simulink model "s7_template_extra"  (R2023a)
settings: Solver=ode4  StartTime=0.0  StopTime=inf  FixedStep=P_sim_dt  RelTol=1e-3
InitFcn:
  | s6_data
values from neighbouring files (symbols this model uses):
  breakslen = varargin{1}    [mbc_ppval.m]
  P_cx_k = 1    [s6_data.m]
  P_p_Bf = 0.7    [p_mad_car.m]
  P_p_Br = 0.7    [p_mad_car.m]
  P_p_Cf = 2    [p_mad_car.m]
  P_p_Cr = 2    [p_mad_car.m]
  P_p_delta_max = 21.58/180*pi    (= 0.37664205258)    [p_mad_car.m]
  P_p_Df = 2    [p_mad_car.m]
  P_p_Dr = 2.5    [p_mad_car.m]
  P_p_Ef = -0.1    [p_mad_car.m]
  P_p_Er = -0.05    [p_mad_car.m]
  P_p_J = 192e-6    (= 0.000192)    [p_mad_car.m]
  P_p_k = 2.51    [p_mad_car.m]
  P_p_kr = 0.344014    [s6_data.m]
  P_p_l = abs(P_p_frontaxle_1 + P_p_rearaxle_1)    [p_mad_car.m]
  P_p_lf = P_p_frontaxle_1    (= 0.05)    [p_mad_car.m]
  P_p_lr = P_p_rearaxle_1    (= 0.049)    [p_mad_car.m]
  P_p_m = 132e-3    (= 0.132)    [p_mad_car.m]
  P_p_T = 316e-3    (= 0.316)    [p_mad_car.m]
  P_p_TA = 0.02    [s6_data.m]
  P_p_Ti = 0.246830    (= 0.24683)    [s6_data.m]
  P_p_Tt = P_p_uTt + P_p_output_Tt    (= 0.1)    [p_mad_car.m]
  P_w_breakslen = uint32(length(path.points))    [s6_data.m]
  P_w_coefs = zeros(SPLINE.Elements(3).Dimensions)    [s6_data.m]
  P_w_points = zeros(SPLINE.Elements(2).Dimensions)    [s6_data.m]
  P_w_segments = uint32(zeros(SPLINE.Elements(4).Dimensions))    [s6_data.m]
  points = [ p.x + x ;      center1 + sign(t.xe) * r * cos(p.psi - pi/2 + sign(t.xe) * x / t.r) ;      center2 + sign(t.xe) * r * sin(p.psi - pi/2 + sign(t.xe) * x / t.r) ]    [mbc_circle_get_points.m]    (also in mbc_clothoid_get_points.m = [ p.x + x ;      s1;      s2]; mbc_spline_create.m = [ points(:, 1:end-1) [ points(1, end); points(2:3, 1) ] ]; mbc_straight_get_points.m = [ p.x + x ;      p.s1 + cpsi * x + (alpha - 0.5) * t.w * cos)
undefined symbols (not defined in the file or in its folder): coefs, DiscIntNeverNeededParam, Display, mad_lib_template, mbc_car_display, P_p_s1_start, P_p_s2_start, P_p_Tw, periodic, segments
settings Model: Creator=hmekiedj  LastModifiedBy=aaron
settings SolverCC: AlgebraicLoopSolver=TrustRegion
settings DataIOCC: ReturnWorkspaceOutputs=off
settings OptimizationCC: BlockReduction=off  DefaultParameterBehavior=Inlined  BufferReuse=off
settings DebuggingCC: SignalInfNanChecking=warning  UnconnectedInputMsg=warning  UnconnectedOutputMsg=warning  UnconnectedLineMsg=warning  ArithmeticOperatorsInVariantConditions=warning
settings ModelReferenceCC: EnableRefExpFcnMdlSchedulingChecks=on
settings SFSimCC: SimUseLocalCustomCode=off  CustomCodeUndefinedFunction=UseInterfaceOnly
settings RTWCC: RTWUseLocalCustomCode=off
settings CodeAppCC: StateflowObjectComments=on

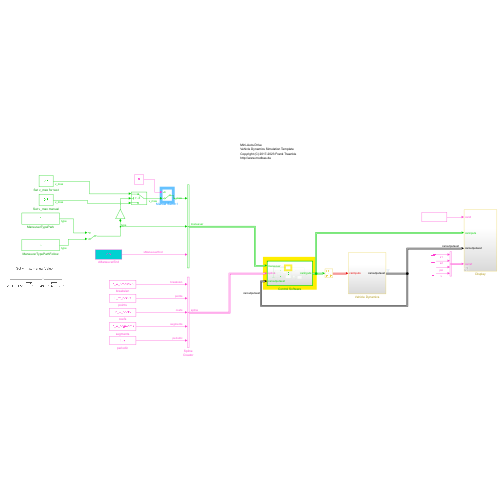
[thumbnail: Simulink's stored preview of the top-level diagram]
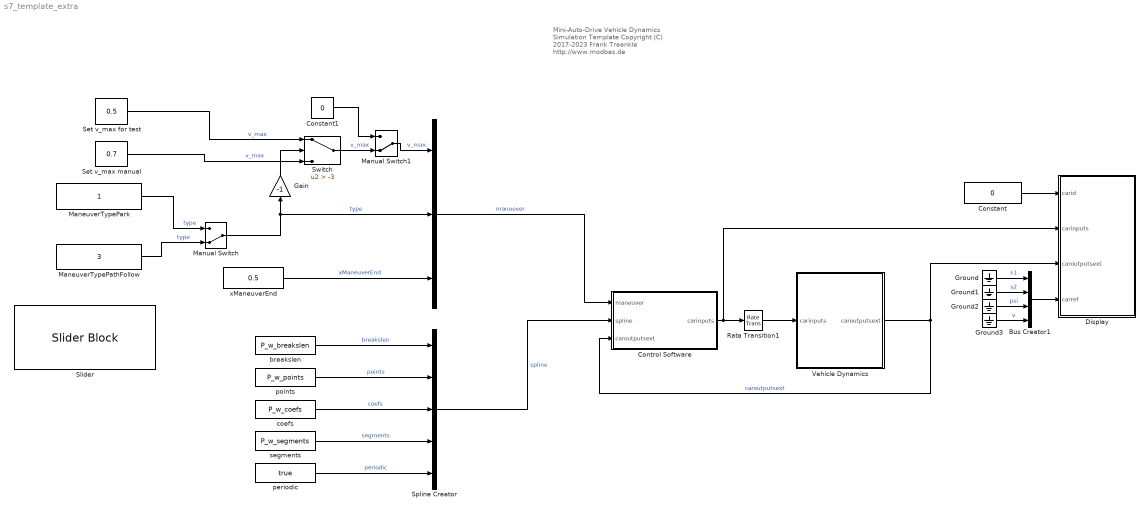
== system s7_template_extra ==
  note: Mini-Auto-Drive
      | Vehicle Dynamics Simulation Template
      | Copyright (C) 2017-2023 Frank Traenkle
      | http://www.modbas.de
  " " : BusCreator  Inputs=3
  Bus Creator1 : BusCreator  Inputs=4
  Constant : Constant  Value=0
  Constant1 : Constant  Value=0
  Control Software : Subsystem  TreatAsAtomicUnit=on  SystemSampleTime=P_p_TA
  Display : Subsystem  AncestorBlock=mad_lib_template/Display
      settings: LibrarySourceBlock=mad_lib_template/Display
  Gain : Gain  Gain=-1
  Ground{,1..3} (4 alike) : Ground
  ManeuverTypePark : Constant  SampleTime=-1
  ManeuverTypePathFollow : Constant  Value=3  SampleTime=-1
  Manual Switch : ManualSwitch  CurrentSetting=0
  Manual Switch1 : ManualSwitch  CurrentSetting=0
  Rate Transition1 : RateTransition
  Set v_max for test : Constant  Value=0.5  SampleTime=-1
  Set v_max manual : Constant  Value=0.7  SampleTime=-1
  Slider : SliderBlock  ScaleMin=-2.51  ScaleMax=2.51
  Spline Creator : BusCreator  Inputs=breakslen,points,coefs,segments,periodic  OutDataTypeStr=Bus: SPLINE
  Switch : Switch  Criteria=u2 > Threshold  Threshold=-3  SaturateOnIntegerOverflow=off  InputSameDT=off
  Vehicle Dynamics : Subsystem
  breakslen : Constant  Value=P_w_breakslen
  coefs : Constant  Value=P_w_coefs
  periodic : Constant  Value=true
  points : Constant  Value=P_w_points
  segments : Constant  Value=P_w_segments
  xManeuverEnd : Constant  Value=0.5
  wires:
  Bus Creator1/1 -> Display/4(carref)
  Ground/1 -> Bus Creator1/1  "s1"
  Ground1/1 -> Bus Creator1/2  "s2"
  Ground2/1 -> Bus Creator1/3  "psi"
  Ground3/1 -> Bus Creator1/4  "v"
  Vehicle Dynamics/1(caroutputsext) -> Display/3(caroutputsext), Control Software/3(caroutputsext)  "caroutputsext"
  Rate Transition1/1 -> Vehicle Dynamics/1(carinputs)
  Constant/1 -> Display/1(carid)
  Control Software/1(carinputs) -> Display/2(carinputs), Rate Transition1/1
  " "/1 -> Control Software/1(maneuver)  "manuever"
  xManeuverEnd/1 -> " "/3  "xManeuverEnd"
  ManeuverTypePathFollow/1 -> Manual Switch/2  "type"
  ManeuverTypePark/1 -> Manual Switch/1  "type"
  Manual Switch/1 -> " "/2, Gain/1  "type"
  Manual Switch1/1 -> " "/1  "v_max"
  Gain/1 -> Switch/2
  Set v_max for test/1 -> Switch/1  "v_max"
  Set v_max manual/1 -> Switch/3  "v_max"
  breakslen/1 -> Spline Creator/1  "breakslen"
  points/1 -> Spline Creator/2  "points"
  coefs/1 -> Spline Creator/3  "coefs"
  segments/1 -> Spline Creator/4  "segments"
  periodic/1 -> Spline Creator/5  "periodic"
  Spline Creator/1 -> Control Software/2(spline)  "spline"
  Switch/1 -> Manual Switch1/2  "v_max"
  Constant1/1 -> Manual Switch1/1

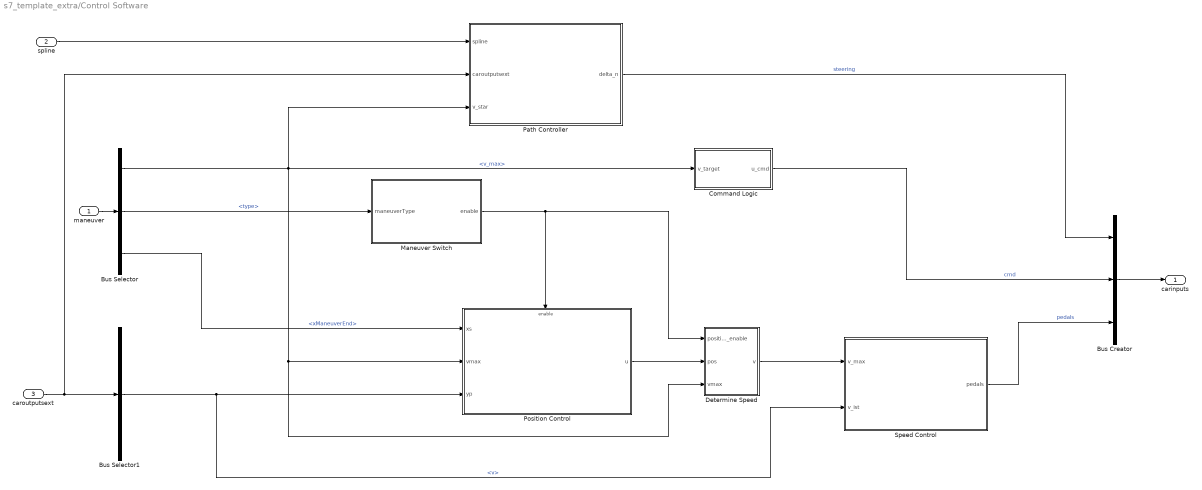
== system s7_template_extra/Control Software ==
  maneuver : Inport
  spline : Inport  Port=2
  caroutputsext : Inport  Port=3
  Bus Creator : BusCreator  Inputs=3
  Bus Selector : BusSelector  OutputSignals=v_max,type,xManeuverEnd
  Bus Selector1 : BusSelector  OutputSignals=v
  Command Logic : MATLAB Function  TreatAsAtomicUnit=on
  Determine Speed : MATLAB Function  TreatAsAtomicUnit=on
  Maneuver Switch : MATLAB Function  TreatAsAtomicUnit=on
  Path Controller : Subsystem
  Position Control : Subsystem
  Speed Control : Subsystem
  carinputs : Outport
  wires:
  maneuver/1 -> Bus Selector/1
  caroutputsext/1 -> Bus Selector1/1, Path Controller/2(caroutputsext)
  Bus Selector1/1 -> Speed Control/2(v_ist), Position Control/3(yp)  "<v>"
  Bus Creator/1 -> carinputs/1
  Speed Control/1(pedals) -> Bus Creator/3  "pedals"
  Bus Selector/1 -> Determine Speed/3(vmax), Position Control/2(vmax), Path Controller/3(v_star), Command Logic/1(v_target)  "<v_max>"
  Bus Selector/2 -> Maneuver Switch/1(maneuverType)  "<type>"
  Bus Selector/3 -> Position Control/1(xs)  "<xManeuverEnd>"
  Position Control/1(u) -> Determine Speed/2(pos)
  Determine Speed/1(v) -> Speed Control/1(v_max)
  Maneuver Switch/1(enable) -> Position Control/Enable, Determine Speed/1(position_enable)
  Command Logic/1(u_cmd) -> Bus Creator/2  "cmd"
  spline/1 -> Path Controller/1(spline)
  Path Controller/1(delta_n) -> Bus Creator/1  "steering"

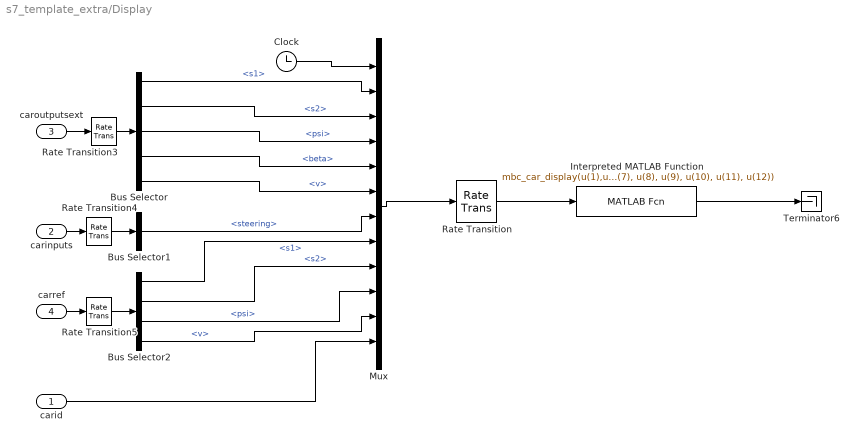
== system s7_template_extra/Display ==
  carid : Inport
  carinputs : Inport  Port=2
  caroutputsext : Inport  Port=3
  carref : Inport  Port=4
  Bus Selector : BusSelector  OutputSignals=s1,s2,psi,beta,v
  Bus Selector1 : BusSelector  OutputSignals=steering
  Bus Selector2 : BusSelector  OutputSignals=s1,s2,psi,v
  Clock : Clock
  Interpreted MATLAB Function : MATLABFcn  MATLABFcn=mbc_car_display(u(1),u(2),u(3),u(4),u(5), u(6), u(7), u(8), u(9), u(10), u(11), u(12))
  Mux : Mux  Inputs=12
  Rate Transition : RateTransition  OutPortSampleTime=P_display_dt
  Rate Transition3 : RateTransition
  Rate Transition4 : RateTransition
  Rate Transition5 : RateTransition
  Terminator6 : Terminator
  wires:
  caroutputsext/1 -> Rate Transition3/1
  Interpreted MATLAB Function/1 -> Terminator6/1
  Mux/1 -> Rate Transition/1
  Rate Transition/1 -> Interpreted MATLAB Function/1
  Clock/1 -> Mux/1
  Bus Selector/1 -> Mux/2  "<s1>"
  Bus Selector/2 -> Mux/3  "<s2>"
  Bus Selector/3 -> Mux/4  "<psi>"
  carinputs/1 -> Rate Transition4/1
  Bus Selector1/1 -> Mux/7  "<steering>"
  Bus Selector/4 -> Mux/5  "<beta>"
  Bus Selector/5 -> Mux/6  "<v>"
  carref/1 -> Rate Transition5/1
  Bus Selector2/4 -> Mux/11  "<v>"
  Bus Selector2/3 -> Mux/10  "<psi>"
  Bus Selector2/2 -> Mux/9  "<s2>"
  Bus Selector2/1 -> Mux/8  "<s1>"
  carid/1 -> Mux/12
  Rate Transition4/1 -> Bus Selector1/1
  Rate Transition3/1 -> Bus Selector/1
  Rate Transition5/1 -> Bus Selector2/1

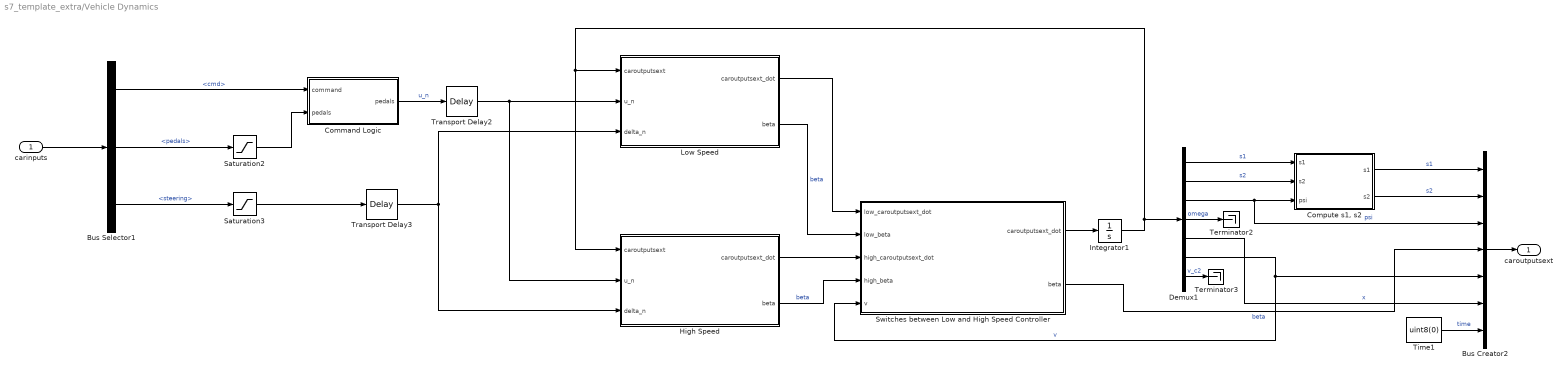
== system s7_template_extra/Vehicle Dynamics ==
  carinputs : Inport
  Bus Creator2 : BusCreator  Inputs=7  OutDataTypeStr=Bus: CAROUTPUTSEXT
  Bus Selector1 : BusSelector  OutputSignals=cmd,pedals,steering
  Command Logic : MATLAB Function  TreatAsAtomicUnit=on
  "Compute s1, s2" : MATLAB Function  TreatAsAtomicUnit=on
  Demux1 : Demux  Outputs=7
  High Speed : Subsystem
  Integrator1 : Integrator  InitialCondition=[P_p_s1_start; P_p_s2_start; 0; 0; 0; 0; 0]
  Low Speed : Subsystem
  Saturation2 : Saturate  UpperLimit=1  LowerLimit=-1
  Saturation3 : Saturate  UpperLimit=1  LowerLimit=-1
  Switches between Low and High Speed Controller : MATLAB Function  TreatAsAtomicUnit=on
  Terminator2 : Terminator
  Terminator3 : Terminator
  Time1 : Constant  Value=uint8(0)
  Transport Delay2 : TransportDelay  DelayTime=P_p_Tt
  Transport Delay3 : TransportDelay  DelayTime=P_p_Tt
  caroutputsext : Outport  VectorParamsAs1DForOutWhenUnconnected=off
  wires:
  Transport Delay3/1 -> Low Speed/3(delta_n), High Speed/3(delta_n)
  Saturation3/1 -> Transport Delay3/1
  Bus Selector1/1 -> Command Logic/1(command)  "<cmd>"
  Command Logic/1(pedals) -> Transport Delay2/1  "u_n"
  Bus Selector1/2 -> Saturation2/1  "<pedals>"
  carinputs/1 -> Bus Selector1/1
  Low Speed/1(caroutputsext_dot) -> Switches between Low and High Speed Controller/1(low_caroutputsext_dot)
  Saturation2/1 -> Command Logic/2("pedals ")
  Transport Delay2/1 -> Low Speed/2(u_n), High Speed/2(u_n)
  High Speed/2(beta) -> Switches between Low and High Speed Controller/4(high_beta)  "beta"
  Low Speed/2(beta) -> Switches between Low and High Speed Controller/2(low_beta)  "beta"
  Bus Selector1/3 -> Saturation3/1  "<steering>"
  High Speed/1(caroutputsext_dot) -> Switches between Low and High Speed Controller/3(high_caroutputsext_dot)
  Switches between Low and High Speed Controller/1(caroutputsext_dot) -> Integrator1/1
  Integrator1/1 -> High Speed/1(caroutputsext), Low Speed/1(caroutputsext), Demux1/1
  Demux1/7 -> Terminator3/1  "v_c2"
  Demux1/6 -> Switches between Low and High Speed Controller/5(v), Bus Creator2/5  "v"
  Demux1/3 -> Bus Creator2/3, "Compute s1, s2"/3(psi)  "psi"
  Time1/1 -> Bus Creator2/7  "time"
  Demux1/4 -> Terminator2/1  "omega"
  Bus Creator2/1 -> caroutputsext/1
  Demux1/1 -> "Compute s1, s2"/1("s1 ")  "s1"
  Demux1/2 -> "Compute s1, s2"/2("s2 ")  "s2"
  "Compute s1, s2"/1(s1) -> Bus Creator2/1  "s1"
  "Compute s1, s2"/2(s2) -> Bus Creator2/2  "s2"
  Switches between Low and High Speed Controller/2(beta) -> Bus Creator2/4  "beta"
  Demux1/5 -> Bus Creator2/6  "x"

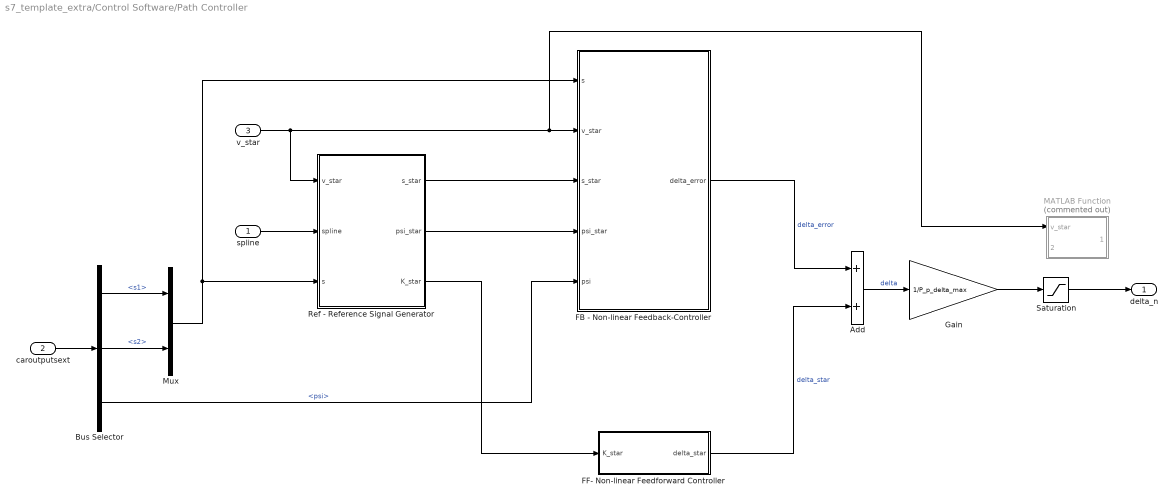
== system s7_template_extra/Control Software/Path Controller ==
  spline : Inport
  caroutputsext : Inport  Port=2
  v_star : Inport  Port=3
  Add : Sum
  Bus Selector : BusSelector  OutputSignals=s1,s2,psi
  FB - Non-linear Feedback-Controller : Subsystem
  FF- Non-linear Feedforward Controller : MATLAB Function  TreatAsAtomicUnit=on
  Gain : Gain  Gain=1/P_p_delta_max
  MATLAB Function : MATLAB Function  Commented=on  TreatAsAtomicUnit=on
  Mux : Mux  Inputs=2
  Ref - Reference Signal Generator : Subsystem
  Saturation : Saturate  UpperLimit=1  LowerLimit=-1
  delta_n : Outport
  wires:
  FF- Non-linear Feedforward Controller/1(delta_star) -> Add/2  "delta_star"
  FB - Non-linear Feedback-Controller/1(delta_error) -> Add/1  "delta_error"
  Add/1 -> Gain/1  "delta"
  v_star/1 -> MATLAB Function/1(v_star), FB - Non-linear Feedback-Controller/2(v_star), Ref - Reference Signal Generator/1(v_star)
  spline/1 -> Ref - Reference Signal Generator/2(spline)
  Ref - Reference Signal Generator/3(K_star) -> FF- Non-linear Feedforward Controller/1(K_star)
  Ref - Reference Signal Generator/2(psi_star) -> FB - Non-linear Feedback-Controller/4(psi_star)
  Ref - Reference Signal Generator/1(s_star) -> FB - Non-linear Feedback-Controller/3(s_star)
  Bus Selector/3 -> FB - Non-linear Feedback-Controller/5(psi)  "<psi>"
  caroutputsext/1 -> Bus Selector/1
  Bus Selector/1 -> Mux/1  "<s1>"
  Bus Selector/2 -> Mux/2  "<s2>"
  Mux/1 -> Ref - Reference Signal Generator/3(s), FB - Non-linear Feedback-Controller/1(s)
  Saturation/1 -> delta_n/1
  Gain/1 -> Saturation/1

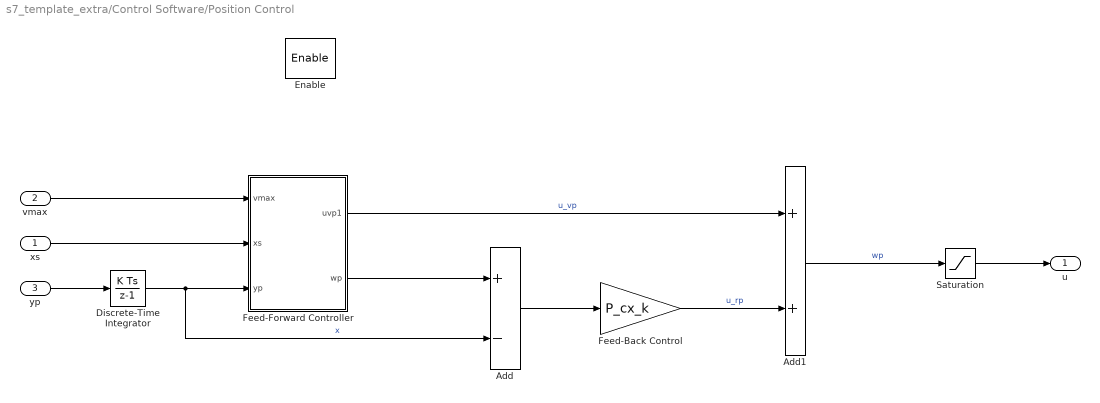
== system s7_template_extra/Control Software/Position Control ==
  xs : Inport
  vmax : Inport  Port=2
  yp : Inport  Port=3
  Enable : EnablePort  StatesWhenEnabling=reset
  Add : Sum  Inputs=+-
  Add1 : Sum
  Discrete-Time Integrator : DiscreteIntegrator  SampleTime=-1  ICPrevOutput=DiscIntNeverNeededParam  ICPrevScaledInput=DiscIntNeverNeededParam
  Feed-Back Control : Gain  Gain=P_cx_k
  Feed-Forward Controller : Subsystem
  Saturation : Saturate  UpperLimit=1  LowerLimit=-1
  u : Outport
  wires:
  Feed-Forward Controller/2(wp) -> Add/1
  Add/1 -> Feed-Back Control/1
  Add1/1 -> Saturation/1  "wp"
  Saturation/1 -> u/1
  Feed-Back Control/1 -> Add1/2  "u_rp"
  Feed-Forward Controller/1(uvp1) -> Add1/1  "u_vp"
  xs/1 -> Feed-Forward Controller/2(xs)
  vmax/1 -> Feed-Forward Controller/1(vmax)
  yp/1 -> Discrete-Time Integrator/1
  Discrete-Time Integrator/1 -> Add/2, Feed-Forward Controller/3(yp)  "x"

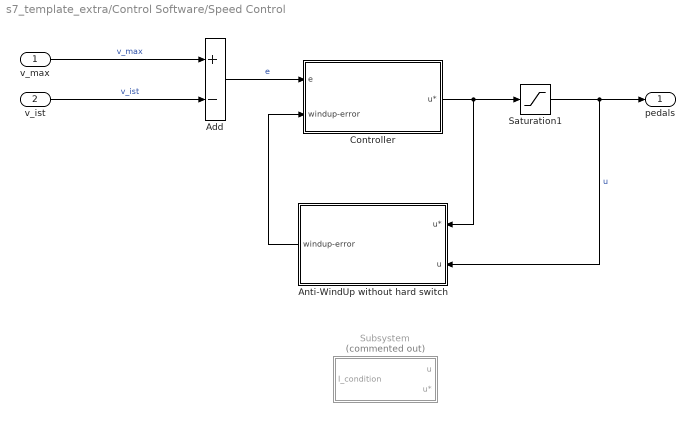
== system s7_template_extra/Control Software/Speed Control ==
  v_max : Inport
  v_ist : Inport  Port=2
  Add : Sum  Inputs=+-
  Anti-WindUp without hard switch : Subsystem
  Controller : Subsystem
  Saturation1 : Saturate  UpperLimit=1  LowerLimit=-1
  Subsystem : Subsystem  Commented=on
  pedals : Outport
  wires:
  v_max/1 -> Add/1  "v_max"
  v_ist/1 -> Add/2  "v_ist"
  Add/1 -> Controller/1(e)  "e"
  Controller/1(u*) -> Anti-WindUp without hard switch/1(u*), Saturation1/1
  Saturation1/1 -> pedals/1, Anti-WindUp without hard switch/2(u)  "u"
  Anti-WindUp without hard switch/1(windup-error) -> Controller/2(windup-error)

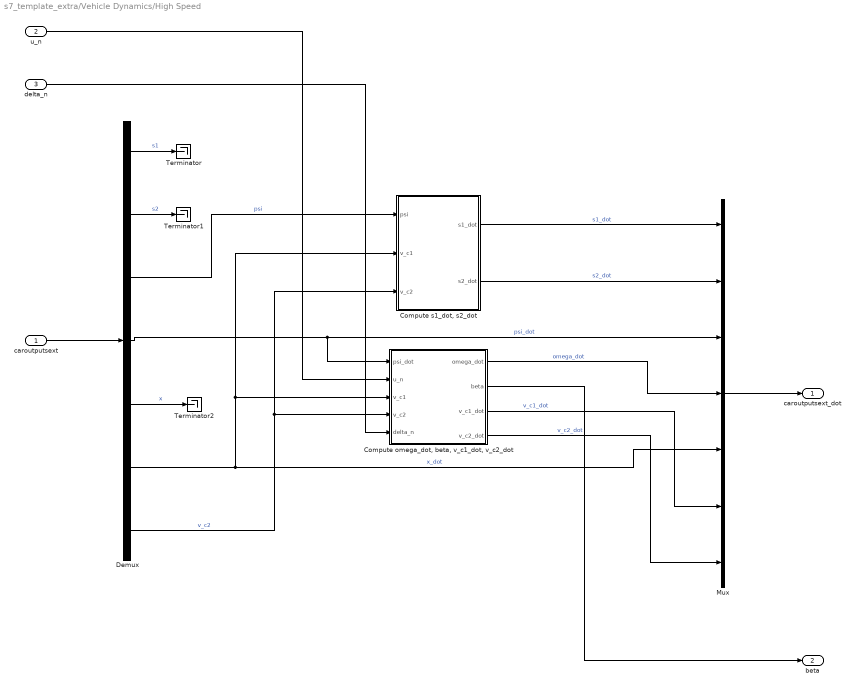
== system s7_template_extra/Vehicle Dynamics/High Speed ==
  caroutputsext : Inport
  u_n : Inport  Port=2
  delta_n : Inport  Port=3
  "Compute omega_dot, beta, v_c1_dot, v_c2_dot" : MATLAB Function  TreatAsAtomicUnit=on
  "Compute s1_dot, s2_dot" : MATLAB Function  TreatAsAtomicUnit=on
  Demux : Demux  Outputs=7
  Mux : Mux  Inputs=7
  Terminator : Terminator
  Terminator1 : Terminator
  Terminator2 : Terminator
  caroutputsext_dot : Outport
  beta : Outport  Port=2
  wires:
  Mux/1 -> caroutputsext_dot/1
  "Compute s1_dot, s2_dot"/2(s2_dot) -> Mux/2  "s2_dot"
  u_n/1 -> "Compute omega_dot, beta, v_c1_dot, v_c2_dot"/2(u_n)
  Demux/1 -> Terminator/1  "s1"
  Demux/2 -> Terminator1/1  "s2"
  Demux/5 -> Terminator2/1  "x"
  Demux/7 -> "Compute omega_dot, beta, v_c1_dot, v_c2_dot"/4(v_c2), "Compute s1_dot, s2_dot"/3(v_c2)  "v_c2"
  delta_n/1 -> "Compute omega_dot, beta, v_c1_dot, v_c2_dot"/5(delta_n)
  Demux/3 -> "Compute s1_dot, s2_dot"/1(psi)  "psi"
  Demux/4 -> "Compute omega_dot, beta, v_c1_dot, v_c2_dot"/1(psi_dot), Mux/3  "psi_dot"
  caroutputsext/1 -> Demux/1
  Demux/6 -> Mux/5, "Compute omega_dot, beta, v_c1_dot, v_c2_dot"/3(v_c1), "Compute s1_dot, s2_dot"/2(v_c1)  "x_dot"
  "Compute s1_dot, s2_dot"/1(s1_dot) -> Mux/1  "s1_dot"
  "Compute omega_dot, beta, v_c1_dot, v_c2_dot"/1(omega_dot) -> Mux/4  "omega_dot"
  "Compute omega_dot, beta, v_c1_dot, v_c2_dot"/3(v_c1_dot) -> Mux/6  "v_c1_dot"
  "Compute omega_dot, beta, v_c1_dot, v_c2_dot"/2(beta) -> beta/1
  "Compute omega_dot, beta, v_c1_dot, v_c2_dot"/4(v_c2_dot) -> Mux/7  "v_c2_dot"

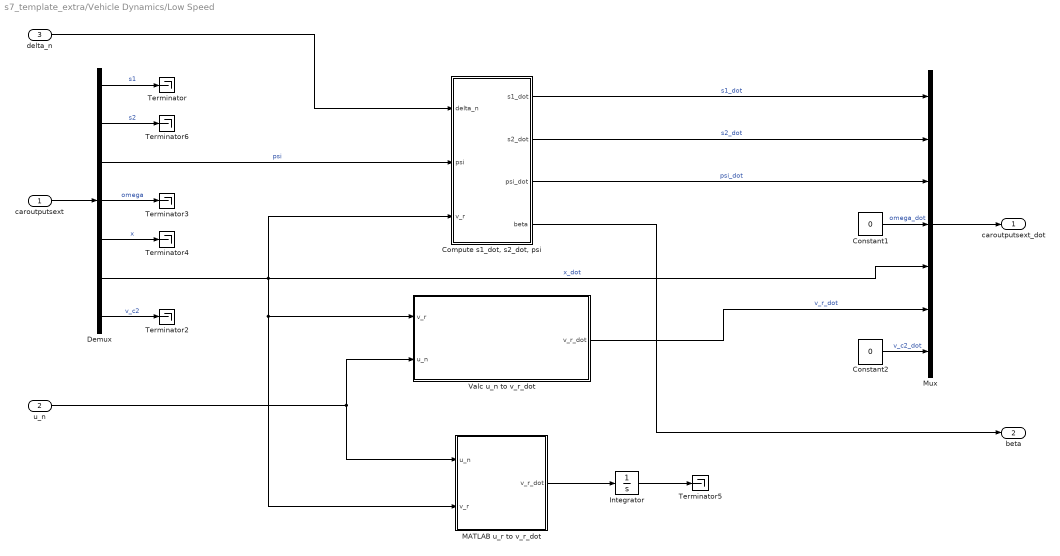
== system s7_template_extra/Vehicle Dynamics/Low Speed ==
  caroutputsext : Inport
  u_n : Inport  Port=2
  delta_n : Inport  Port=3
  "Compute s1_dot, s2_dot, psi" : MATLAB Function  TreatAsAtomicUnit=on
  Constant1 : Constant  Value=0
  Constant2 : Constant  Value=0
  Demux : Demux  Outputs=7
  Integrator : Integrator
  MATLAB u_r to v_r_dot : MATLAB Function  TreatAsAtomicUnit=on
  Mux : Mux  Inputs=7
  Terminator{,2..6} (6 alike) : Terminator
  Valc u_n to v_r_dot : Subsystem
  caroutputsext_dot : Outport
  beta : Outport  Port=2
  wires:
  caroutputsext/1 -> Demux/1
  Mux/1 -> caroutputsext_dot/1
  Demux/3 -> "Compute s1_dot, s2_dot, psi"/2(psi)  "psi"
  delta_n/1 -> "Compute s1_dot, s2_dot, psi"/1(delta_n)
  "Compute s1_dot, s2_dot, psi"/1(s1_dot) -> Mux/1  "s1_dot"
  "Compute s1_dot, s2_dot, psi"/2(s2_dot) -> Mux/2  "s2_dot"
  Demux/6 -> "Compute s1_dot, s2_dot, psi"/3(v_r), Mux/5, MATLAB u_r to v_r_dot/2(v_r), Valc u_n to v_r_dot/1(v_r)  "x_dot"
  u_n/1 -> MATLAB u_r to v_r_dot/1(u_n), Valc u_n to v_r_dot/2(u_n)
  Demux/5 -> Terminator4/1  "x"
  Constant1/1 -> Mux/4  "omega_dot"
  Demux/4 -> Terminator3/1  "omega"
  Demux/7 -> Terminator2/1  "v_c2"
  MATLAB u_r to v_r_dot/1(v_r_dot) -> Integrator/1
  Valc u_n to v_r_dot/1(v_r_dot) -> Mux/6  "v_r_dot"
  Integrator/1 -> Terminator5/1
  Demux/1 -> Terminator/1  "s1"
  Demux/2 -> Terminator6/1  "s2"
  "Compute s1_dot, s2_dot, psi"/3(psi_dot) -> Mux/3  "psi_dot"
  "Compute s1_dot, s2_dot, psi"/4(beta) -> beta/1
  Constant2/1 -> Mux/7  "v_c2_dot"

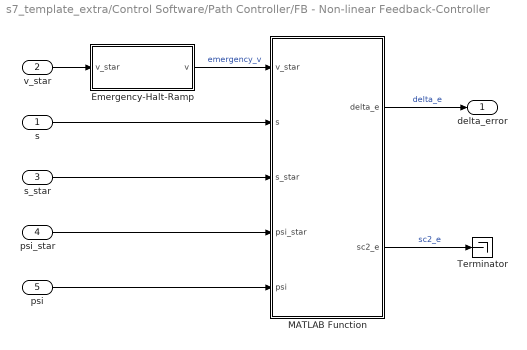
== system s7_template_extra/Control Software/Path Controller/FB - Non-linear Feedback-Controller ==
  s : Inport
  v_star : Inport  Port=2
  s_star : Inport  Port=3
  psi_star : Inport  Port=4
  psi : Inport  Port=5
  Emergency-Halt-Ramp : Subsystem
  MATLAB Function : MATLAB Function  TreatAsAtomicUnit=on
  Terminator : Terminator
  delta_error : Outport
  wires:
  MATLAB Function/1(delta_e) -> delta_error/1  "delta_e"
  v_star/1 -> Emergency-Halt-Ramp/1(v_star)
  psi_star/1 -> MATLAB Function/4(psi_star)
  psi/1 -> MATLAB Function/5(psi)
  s/1 -> MATLAB Function/2(s)
  s_star/1 -> MATLAB Function/3(s_star)
  Emergency-Halt-Ramp/1(v) -> MATLAB Function/1(v_star)  "emergency_v"
  MATLAB Function/2(sc2_e) -> Terminator/1  "sc2_e"

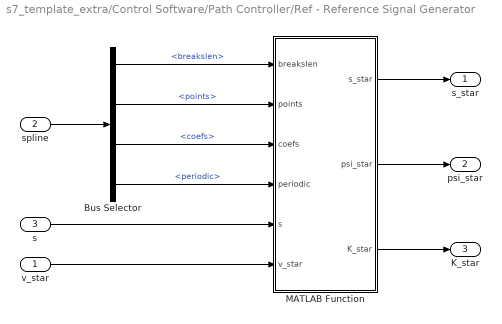
== system s7_template_extra/Control Software/Path Controller/Ref - Reference Signal Generator ==
  v_star : Inport
  spline : Inport  Port=2
  s : Inport  Port=3
  Bus Selector : BusSelector  OutputSignals=breakslen,points,coefs,periodic
  MATLAB Function : MATLAB Function  TreatAsAtomicUnit=on
  s_star : Outport
  psi_star : Outport  Port=2
  K_star : Outport  Port=3
  wires:
  v_star/1 -> MATLAB Function/6(v_star)
  MATLAB Function/1(s_star) -> s_star/1
  MATLAB Function/2(psi_star) -> psi_star/1
  MATLAB Function/3(K_star) -> K_star/1
  spline/1 -> Bus Selector/1
  Bus Selector/1 -> MATLAB Function/1(breakslen)  "<breakslen>"
  Bus Selector/3 -> MATLAB Function/3(coefs)  "<coefs>"
  Bus Selector/2 -> MATLAB Function/2(points)  "<points>"
  Bus Selector/4 -> MATLAB Function/4(periodic)  "<periodic>"
  s/1 -> MATLAB Function/5(s)

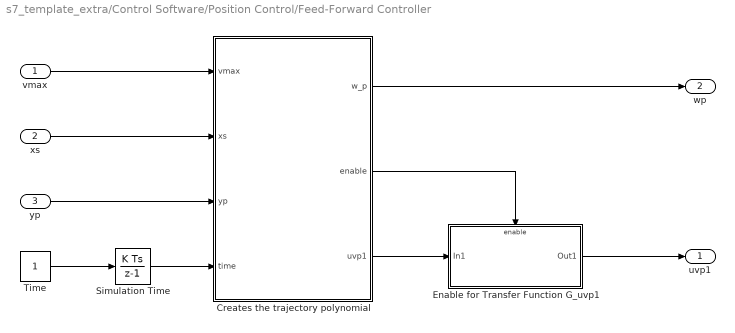
== system s7_template_extra/Control Software/Position Control/Feed-Forward Controller ==
  vmax : Inport
  xs : Inport  Port=2
  yp : Inport  Port=3
  Creates the trajectory polynomial : MATLAB Function  TreatAsAtomicUnit=on
  "Enable for Transfer Function G_uvp1 " : Subsystem
  Simulation Time : DiscreteIntegrator  SampleTime=-1  ICPrevOutput=DiscIntNeverNeededParam  ICPrevScaledInput=DiscIntNeverNeededParam
  Time : Constant
  uvp1 : Outport
  wp : Outport  Port=2
  wires:
  yp/1 -> Creates the trajectory polynomial/3(yp)
  vmax/1 -> Creates the trajectory polynomial/1(vmax)
  xs/1 -> Creates the trajectory polynomial/2(xs)
  Creates the trajectory polynomial/1(w_p) -> wp/1
  Simulation Time/1 -> Creates the trajectory polynomial/4(time)
  Time/1 -> Simulation Time/1
  Creates the trajectory polynomial/3(uvp1) -> "Enable for Transfer Function G_uvp1 "/1(In1)
  "Enable for Transfer Function G_uvp1 "/1(Out1) -> uvp1/1
  Creates the trajectory polynomial/2(enable) -> "Enable for Transfer Function G_uvp1 "/Enable

== system s7_template_extra/Control Software/Speed Control/Anti-WindUp without hard switch ==
  note: Anti-Wind-Up without hard switch
  u* : Inport
  u : Inport  Port=2
  Gain : Gain  Gain=0.1
  Sum : Sum  Inputs=|-+
  Unit Delay : UnitDelay  SampleTime=-1  HasFrameUpgradeWarning=on
  windup-error : Outport
  wires:
  u*/1 -> Sum/1
  u/1 -> Sum/2
  Sum/1 -> Gain/1
  Gain/1 -> Unit Delay/1
  Unit Delay/1 -> windup-error/1

== system s7_template_extra/Control Software/Speed Control/Controller ==
  e : Inport
  windup-error : Inport  Port=2
  Add : Sum
  Add1 : Sum  Inputs=+++
  Delay : Delay  DelayLength=1  SampleTime=0.02
  Gain : Gain  Gain=P_p_kr
  Gain1 : Gain  Gain=(P_p_kr*P_p_TA) / P_p_Ti
  u* : Outport
  wires:
  Add/1 -> u*/1  "u*"
  Gain/1 -> Add/1  "u_pk"
  e/1 -> Gain/1, Gain1/1
  Gain1/1 -> Add1/2
  Delay/1 -> Add1/1
  Add1/1 -> Delay/1, Add/2  "u_ik"
  windup-error/1 -> Add1/3

== system s7_template_extra/Control Software/Speed Control/Subsystem ==
  u : Inport
  u* : Inport  Port=2
  MATLAB Function : MATLAB Function  TreatAsAtomicUnit=on
  I_condition : Outport
  wires:
  MATLAB Function/1(y) -> I_condition/1
  u/1 -> MATLAB Function/1(u)
  u*/1 -> MATLAB Function/2(u_stern)

== system s7_template_extra/Vehicle Dynamics/Low Speed/Valc u_n to v_r_dot ==
  v_r : Inport
  u_n : Inport  Port=2
  Add : Sum  Inputs=+-
  Gain1 : Gain  Gain=(P_p_k/P_p_T)
  Gain2 : Gain  Gain=1/P_p_T
  v_r_dot : Outport
  wires:
  Gain2/1 -> Add/2
  u_n/1 -> Gain1/1
  Gain1/1 -> Add/1
  Add/1 -> v_r_dot/1  "v_r_dot"
  v_r/1 -> Gain2/1

== system s7_template_extra/Control Software/Path Controller/FB - Non-linear Feedback-Controller/Emergency-Halt-Ramp ==
  v_star : Inport
  Discrete Transfer Fcn : DiscreteTransferFcn  Commented=through  Denominator=[1 1]
  Generate_ramp : MATLAB Function  TreatAsAtomicUnit=on
  v : Outport
  wires:
  v_star/1 -> Discrete Transfer Fcn/1  "v_star"
  Generate_ramp/1(v) -> v/1
  Discrete Transfer Fcn/1 -> Generate_ramp/1(v_star)  "disc_v_star"

== system s7_template_extra/Control Software/Position Control/Feed-Forward Controller/Enable for Transfer Function G_uvp1  ==
  In1 : Inport
  Enable : EnablePort
  Discrete High-Pass-Filter Gvp1 : DiscreteTransferFcn  Numerator=[2 -2]  Denominator=[(2*P_p_Ti+P_p_T) (P_p_T-2*P_p_Ti)]
  Out1 : Outport
  wires:
  Discrete High-Pass-Filter Gvp1/1 -> Out1/1
  In1/1 -> Discrete High-Pass-Filter Gvp1/1

== matlab function s7_template_extra/Vehicle Dynamics/Switches between Low and High Speed Controller ==
  data: low_caroutputsext_dot input; low_beta input; caroutputsext_dot output; high_caroutputsext_dot input; high_beta input; v input; beta output
function [caroutputsext_dot, beta] = SwitchControllers(low_caroutputsext_dot, low_beta, high_caroutputsext_dot, high_beta, v)
% Switch between low and high speed controllers based on vehicle speed.
%
% This function selects either the low or high speed controller for vehicle dynamics 
% based on the current speed of the vehicle. It outputs the appropriate control 
% parameters and the beta values for the chosen controller.
%
% Syntax:
%   [caroutputsext_dot, beta] = SwitchControllers(low_caroutputsext_dot, low_beta, 
%                                  high_caroutputsext_dot, high_beta, v)
%
% Inputs:
%   low_caroutputsext_dot - Control parameters from the low-speed controller.
%   low_beta             - 'Beta' value from the low-speed controller.
%   high_caroutputsext_dot- Control parameters from the high-speed controller.
%   high_beta            - 'Beta' value from the high-speed controller.
%   v                    - Current speed of the vehicle [m/s].
%
% Outputs:
%   caroutputsext_dot    - Selected control parameters for the vehicle's dynamics.
%   beta                 - 'Beta' value to be used in the next program run, based 
%                          on the selected speed controller.


if v < 0.2
    caroutputsext_dot = low_caroutputsext_dot;
    beta = low_beta;
else
    caroutputsext_dot = high_caroutputsext_dot;
    beta = high_beta;
end

== matlab function s7_template_extra/Vehicle Dynamics/Command Logic ==
  data: command input; pedals input; pedals output
function pedals = DetermineCommand(command, pedals)
% Adjusts pedal values based on the current command mode for vehicle control.
%
% This function interprets and adjusts the pedal values according to the given command mode, 
% ensuring appropriate vehicle motion control. The command decides the driving direction 
% (halt, forward, reverse). The function also handles potential error cases, such as preventing 
% reverse motion when the command is set to move forward, and vice versa.
%
% Syntax:
%   pedals = DetermineCommand(command, pedals)
%
% Inputs:
%   command - Numeric value representing the current driving mode. 
%             0: Halt, 1: Forward, 2: Reverse.
%   pedals  - Pedal input, ranging from -1 to 1, where negative values 
%             suggest reverse motion and positive values indicate forward motion.
%
% Output:
%   pedals  - Adjusted pedal value, which acts as a voltage level for the DC motor, 
%             ensuring the vehicle moves in the correct direction as per the command.

    switch command
        case 0      % CarInputsCmdHalt
            pedals = 0;
        case 1  % CarInputsCmdForward 
            if (pedals < 0)
                pedals = 0;
            end
        case 2  % CarInputsCmdReverse 
            if (pedals > 0)
                pedals = 0;
            end
     end
end

== matlab function s7_template_extra/Control Software/Path Controller/FF- Non-linear Feedforward Controller ==
  data: K_star input; delta_star output; P_p_l parameter
function delta_star = FeedforwardSteering(K_star, P_p_l)
% Calculate steering angle for non-linear feedforward control.
%
% This function computes the steering angle, delta_star, using a non-linear 
% feedforward control approach derived from the vehicle's non-linear yaw dynamics.
% The steering angle is calculated in radians.
%
% Syntax:
%   delta_star = FeedforwardSteering(K_star, P_p_l)
%
% Inputs:
%   K_star - Target path curvature, expressed as the inverse of the radius 
%            of the path (in 1/m).
%   P_p_l  - Wheelbase of the vehicle [m].
%        
% Outputs:
%   delta_star - Calculated steering angle in radians [rad], obtained from the 
%                non-linear feedforward control system.

delta_star = atan(P_p_l * K_star);
end

== matlab function s7_template_extra/Control Software/Path Controller/FB - Non-linear Feedback-Controller/MATLAB Function ==
  data: v_star input; delta_e output; s input; s_star input; psi_star input; psi input; P_p_l parameter; P_p_Tw parameter; sc2_e output
function [delta_e, sc2_e] = FeedbackSteering(v_star, s, s_star, psi_star, psi, P_p_l, P_p_Tw)
% Calculate the steering angle error for feedback control in vehicle dynamics.
%
% This function computes the error in the steering angle, delta_e, as part of a 
% linearized dynamic control system. It integrates a non-linear state controller 
% where the control signal is the steering angle. This angle is used in combination 
% with the output of non-linear feedforward control (FF) as a sum.
%
% Syntax:
%   delta_e = FeedbackSteering(v_star, s, s_star, psi_star, psi, P_p_l, P_p_Tw)
%
% Inputs:
%   v_star   - Target speed of the vehicle [m/s].
%   s        - Position vector of the rear axle [m].
%   s_star   - Point vector on the target track curve [m].
%   psi_star - Reference yaw angle [rad].
%   psi      - Actual yaw angle of the vehicle [rad].
%   P_p_l    - Wheelbase of the vehicle [m].
%   P_p_Tw   - Closed-loop time constant [s].
%        
% Outputs:
%   delta_e  - Error in the steering angle [rad], calculated from the
%              difference between the actual and reference states.

s_e = (s - s_star');        % Calc the difference vector s_e on the normal to the nominal path curve determined with the s_star and position of the Rear axle
n_star = [-sin(psi_star); cos(psi_star)];  % normal vector 

psi_e = psi - psi_star; % calculate the error of the yaw angle with the the reference yaw angle and the the real yaw angle of the vehicle 
sc2_e = s_e' * n_star; % calculate the orthogonal distance sc2_e of the rear axle centre point s to the next point s_star on the target path curve 

% normalize psi_e to [-pi, pi]
psi_e = mod(psi_e + pi, 2*pi) - pi; % psi_e [ rad ]

% Constrain v_star to avoid singularity at v_star = 0
v_e = 0.1; % v_e [ m/s ]
if v_star > v_e || v_star < -v_e
    v_star = v_star;
elseif v_star >= 0 && v_star <= v_e
    v_star = v_e;
elseif v_star >= -v_e && v_star < 0
    v_star = -v_e;
end

delta_e = -(P_p_l / (P_p_Tw^2 * v_star^2)) * sc2_e ...
    - (2*P_p_l / (P_p_Tw * v_star)) * psi_e;

end

== matlab function s7_template_extra/Vehicle Dynamics/High Speed/Compute omega_dot, beta, v_c1_dot, v_c2_dot ==
  data: omega_dot output; beta output; psi_dot input; u_n input; v_c1_dot output; v_c1 input; v_c2 input; delta_n input; P_p_k parameter; P_p_lr parameter; P_p_Bf parameter; P_p_Cf parameter; P_p_Df parameter; P_p_Ef parameter; P_p_Br parameter; P_p_Cr parameter; P_p_Dr parameter; P_p_Er parameter; P_p_T parameter; v_c2_dot output; P_p_m parameter; P_p_lf parameter; P_p_delta_max parameter; P_p_J parameter
function [omega_dot, beta, v_c1_dot, v_c2_dot] = fcn(psi_dot, u_n, v_c1, v_c2, delta_n, ...
    P_p_k, P_p_lr, P_p_Bf, P_p_Cf, P_p_Df, P_p_Ef, P_p_Br, P_p_Cr, P_p_Dr, P_p_Er, ...
    P_p_T, P_p_m, P_p_lf, P_p_delta_max, P_p_J)
% Calculate dynamic vehicle parameters based on control inputs and motion state.
%
% This function computes the angular acceleration of the vehicle (omega_dot), 
% the floating angle (beta), and the longitudinal and lateral components of 
% the center of gravity acceleration (v_c1_dot, v_c2_dot). It uses various 
% vehicle parameters, control inputs, and the current state of motion.
%
% Syntax:
%   [omega_dot, beta, v_c1_dot, v_c2_dot] = fcn(psi_dot, u_n, v_c1, v_c2, delta_n, ...
%       P_p_k, P_p_lr, P_p_Bf, P_p_Cf, P_p_Df, P_p_Ef, P_p_Br, P_p_Cr, P_p_Dr, P_p_Er, ...
%       P_p_T, P_p_m, P_p_lf, P_p_delta_max, P_p_J)
%
% Inputs:
%   psi_dot - Yaw rate [rad/s].
%   u_n - Voltage for the DC motor [V].
%   v_c1 - Longitudinal component of the COG velocity [m/s].
%   v_c2 - Lateral component of the COG velocity [m/s].
%   [List other input parameters with descriptions].
%
% Outputs:
%   omega_dot - Angular acceleration [rad/s^2].
%   beta - Floating angle [rad].
%   v_c1_dot - Longitudinal acceleration of the COG [m/s^2].
%   v_c2_dot - Lateral acceleration of the COG [m/s^2].


delta = P_p_delta_max * delta_n;

if(v_c1 > 0)
    % we will use this equation if the velocity v_c1 is above 0 (v_c1 > 0)
    alpha_r = -atan((v_c2 - P_p_lr * psi_dot) / v_c1);
    alpha_f = -atan((v_c2 + P_p_lf * psi_dot) / v_c1) + delta;
elseif (v_c1 < 0)
    % we will use this equation if the velocity v_c1 is below 0 (v_c1 < 0)
    alpha_r = atan((v_c2 - P_p_lr * psi_dot) / v_c1);
    alpha_f = atan((v_c2 + P_p_lf * psi_dot) / v_c1) - delta;
else
    alpha_r = 0;
    alpha_f = 0;
end

Ff = P_p_Df * sin(P_p_Cf * atan(P_p_Bf * (1 - P_p_Ef) * alpha_f ...
    - P_p_Ef * atan(P_p_Bf * alpha_f)));

Fr = P_p_Dr * sin(P_p_Cr * atan(P_p_Br * (1 - P_p_Er) * alpha_r ...
    - P_p_Er * atan(P_p_Br * alpha_r)));

v_c1_dot = (1/P_p_m) * (-Ff * sin(delta) + P_p_m * v_c2 * psi_dot) ...
    - 1/P_p_T * v_c1 ...
    + (P_p_k/P_p_T) * u_n;

v_c2_dot = (1/P_p_m) * (Ff * cos(delta) + Fr - P_p_m * v_c1 * psi_dot);

beta = atan2(v_c2, v_c1);
omega_dot = (1/P_p_J) * (Ff * P_p_lf * cos(delta) - Fr * P_p_lr);

== matlab function s7_template_extra/Vehicle Dynamics/High Speed/Compute s1_dot, s2_dot ==
  data: psi input; v_c1 input; s1_dot output; v_c2 input; s2_dot output
function [s1_dot, s2_dot] = fcn(psi, v_c1, v_c2)
% Calculate Cartesian components of the center of gravity velocity.
%
% This function computes the Cartesian components (s1_dot and s2_dot) of the 
% center of gravity (COG) velocity of a vehicle based on its yaw angle, and 
% longitudinal and lateral components of the COG velocity. 
%
% Syntax:
%   [s1_dot, s2_dot] = fcn(psi, v_c1, v_c2)
%
% Inputs:
%   psi  - Yaw angle of the vehicle [rad].
%   v_c1 - Longitudinal component of the COG velocity [m/s].
%   v_c2 - Lateral component of the COG velocity [m/s].
%
% Outputs:
%   s1_dot - Speed in the direction of s1 (first Cartesian coordinate of the COG) [m/s].
%   s2_dot - Speed in the direction of s2 (second Cartesian coordinate of the COG) [m/s].


s1_dot = v_c1 * cos(psi) - v_c2 * sin(psi);
s2_dot = v_c1 * sin(psi) + v_c2 * cos(psi);
end

== matlab function s7_template_extra/Vehicle Dynamics/Low Speed/MATLAB u_r to v_r_dot ==
  data: u_n input; v_r input; v_r_dot output; P_p_k parameter; P_p_T parameter
function v_r_dot = fcn(u_n, v_r, P_p_k, P_p_T)

v_r_dot = (-1/P_p_T) * v_r + (P_p_k/P_p_T) * u_n;

== matlab function s7_template_extra/Vehicle Dynamics/Compute s1, s2 ==
  data: s1 input; s1 output size=[1 7]; s2 input; psi input; s2 output size=1; P_p_lr parameter
function [s1, s2] = Computes1s2(s1, s2, psi, P_p_lr)
%CreateCarOutputExt Generate extended car outputs.

% Description:
%   This function computes the extended outputs for the car based on the 
%   previously integrated values of the high or low speed controller, the 
%   slip angle (beta), and rear axle distance (P_p_lr). It calculates 
%   the adjusted lateral and longitudinal positions, orientation, and the
%   other parameters
%
% Inputs:
%   s1 - position in driection of s1 the first cartesian coordinate of the centre of gravity [ m ] 
%   s2 - position in driection of s2 the second cartesian coordinate of the centre of gravity [ m ] 
%   beta - A scalar representing floating angle [ rad ]
%   P_p_lr - A scalar representing distance from COG to rear axle [ m ]
%
% Outputs:
%   s1 - position in driection of s1 the first cartesian coordinate of the centre of gravity [ m ] 
%   s2 - position in driection of s2 the second cartesian coordinate of the centre of gravity [ m ]             

s1 = s1 - cos(psi).*P_p_lr;
s2 = s2 - sin(psi).*P_p_lr;
return

== matlab function s7_template_extra/Vehicle Dynamics/Low Speed/Compute s1_dot, s2_dot, psi ==
  data: s1_dot output; s2_dot output; psi_dot output; beta output; delta_n input; psi input; v_r input; P_p_l parameter; P_p_delta_max parameter; P_p_lr parameter
function [s1_dot, s2_dot, psi_dot, beta] = fcn(delta_n, psi, v_r, P_p_l, P_p_delta_max, P_p_lr)
% Calculate dynamic parameters of a vehicle based on steering and motion inputs.
%
% This function computes the dynamic parameters of the car, including the 
% Cartesian components of the center of gravity velocity, yaw rate, and floating 
% angle. It takes into account the vehicle's steering angle, yaw angle, rear axle 
% speed, and geometrical parameters.
%
% Syntax:
%   [s1_dot, s2_dot, psi_dot, beta] = fcn(delta_n, psi, v_r, P_p_l, P_p_delta_max, P_p_lr)
%
% Inputs:
%   delta_n        - Normalized steering angle [rad].
%   psi            - Yaw angle [rad].
%   v_r            - Speed at the rear axle [m/s].
%   P_p_l          - Wheelbase of the vehicle [m].
%   P_p_delta_max  - Maximum steering angle [rad].
%   P_p_lr         - Distance from center of gravity (COG) to rear axle [m].
%
% Outputs:
%   s1_dot         - Speed in the direction of s1 (first Cartesian coordinate 
%                    of the COG) [m/s].
%   s2_dot         - Speed in the direction of s2 (second Cartesian coordinate 
%                    of the COG) [m/s].
%   psi_dot        - Yaw rate [rad/s].
%   beta           - Floating angle [rad], representing the angle between the 
%                    vehicle's velocity vector and its longitudinal axis.


beta = atan( (P_p_lr/P_p_l) * tan(P_p_delta_max * delta_n));

s1_dot =  (v_r/cos(beta))  * cos(psi + beta);
s2_dot = (v_r/cos(beta)) * sin(psi + beta);

psi_dot = (v_r/P_p_l) * tan(P_p_delta_max * delta_n);

end

== matlab function s7_template_extra/Control Software/Path Controller/MATLAB Function ==
  data: v_star input; delta_n output; delta_n input
function delta_n = fcn(v_star, delta_n)

persistent v_star_old v_star_step;
% v_star = 0
% v_star_old = 1.5

if isempty(v_star_old)
    v_star_old = v_star;
    v_star_step = v_star;
end

range = 0.2;
if v_star == 0 && abs(v_star - v_star_old) > 0.1    % emergency halt
    delta_n = min(max(delta_n, -range), +range); % psi_e [ rad ]        % reduce speed by step size until 0
else
    delta_n = delta_n;   % delta_n is within range

end


if 

y = u;

== matlab function s7_template_extra/Control Software/Path Controller/FB - Non-linear Feedback-Controller/Emergency-Halt-Ramp/Generate_ramp ==
  data: v_star input; v output
function v = Generate_ramp(v_star)
persistent v_star_old v_star_step;
% v_star = 0
% v_star_old = 1.5

if isempty(v_star_old)
    v_star_old = v_star;
    v_star_step = v_star;
end

if v_star == 0 && abs(v_star - v_star_old) > 0.1    % emergency halt
    v = v_star_step - 0.05        % reduce speed by step size until 0
    v_star_step = v;
    v_star_old = v;
else
    v = v_star;   % set v to current target speed
    v_star_step = v_star;
    v_star_old = v_star;    % update v_star_old to current speed
end

== matlab function s7_template_extra/Control Software/Speed Control/Subsystem/MATLAB Function ==
  data: u input; y output; u_stern input
function y = fcn(u, u_stern )


if(u ~= u_stern)
    y = 1;
else
    y = 0;
end

== matlab function s7_template_extra/Control Software/Command Logic ==
  data: v_target input; u_cmd output
function u_cmd = SetCommand(v_target)
% SetCommand Determines the command based on the target velocity.
%
%   u_cmd = SETCOMMAND(v_target) returns a command based on the sign of the
%   target velocity (v_target). If the target velocity is non-negative, the 
%   command for forward motion is set, otherwise the command for reverse 
%   motion is set.
%
%   Inputs:
%       v_target - A scalar value representing the target velocity.
%
%   Outputs:
%       u_cmd - An integer representing the command.
%               1 indicates a forward command ("CarInputsCmdForward").
%               2 indicates a reverse command ("CarInputsCmdReverse").

    if v_target >= 0
        u_cmd = uint8(1);   % "CarInputsCmdForward"
    else
        u_cmd = uint8(2);   % "CarInputsCmdReverse"
    end
end

== matlab function s7_template_extra/Control Software/Position Control/Feed-Forward Controller/Creates the trajectory polynomial ==
  data: vmax input; w_p output; enable output; xs input; yp input; uvp1 output; time input; P_p_Ti parameter; P_p_kr parameter; P_p_k parameter; P_p_T parameter; P_p_Tt parameter
function [w_p, enable, uvp1]= ComputePolynomial(vmax, xs, yp, time, P_p_Ti, P_p_kr, P_p_k, P_p_T, P_p_Tt)
% ComputePolynomial Computes a polynomial trajectory and feedforward control.
%
%   [w_p, enable, uvp1] = ComputePolynomial(vmax, xs, yp, time, P_p_Ti, P_p_kr, 
%   P_p_k, P_p_T, P_p_Tt) computes the polynomial trajectory (w_p) and the 
%   feedforward control (uvp1) given a maximum velocity (vmax), start and 
%   end positions (xs, yp), and current time. The function uses controller 
%   parameters (P_p_Ti, P_p_kr, P_p_k, P_p_T, P_p_Tt) to calculate feedforward 
%   terms. The output 'enable' indicates whether the trajectory is finished.
%
%   The function uses persistent variables to retain the coefficients and 
%   final time (te) across function calls.
%
%   Inputs:
%       vmax - Maximum velocity for the polynomial trajectory [ m/s ].
%       xs - Start position for the trajectory [ m ].
%       yp - Current position, used to initialize trajectory on first call [ m ].
%       time - Current time for evaluating the polynomial trajectory [ s ].
%       P_p_Ti - Controller parameter for integral time.
%       P_p_kr - Controller parameter for proportional gain.
%       P_p_k - Controller parameter.
%       P_p_T - Controller parameter for time constant.
%       P_p_Tt - Controller parameter for derivative time.
%
%   Outputs:
%       w_p - The polynomial trajectory at the current time.
%       enable - Boolean flag indicating if the trajectory is still active.
%       uvp1 - The feedforward control term at the current time.

persistent c cff te x0;

% first iteraton step: initialize x0 mit with feedback, 
% then compute coefficients and te 
if isempty(c)
    x0 = yp;

    [c, te] = cd_refpoly_vmax(vmax, x0, xs);
    %te = te + time
    cff = cd_refpoly_ff(c, P_p_k, P_p_T, P_p_Tt, P_p_kr, P_p_Ti);
end

if time >= te     % finished
    enable = false;
    % create polynomial w_p from coefficients
    w_p = polyval(c, te);
    % Compute uvp1 by using cd_refpoly_ff.m function
    uvp1 = polyval(cff, te);
else
    enable = true;
    w_p = polyval(c, time);
    uvp1 = polyval(cff, time);
end

== matlab function s7_template_extra/Control Software/Maneuver Switch ==
  data: maneuverType input; enable output
function enable  = ManeuverSwitch(maneuverType)
% ManeuverSwitch determines the enable state for a maneuver.
%
%   enable = ManeuverSwitch(maneuverType) returns an enable value
%   based on the type of maneuver. The input parameter 'maneuverType' is
%   an integer that identifies the type of maneuver.
%
%   Inputs:
%       maneuverType - An integer that specifies the type of maneuver.
%                      Possible values are:
%                      1: Parking maneuver for longitudinal position control 
%                      3: Path following maneuver for speed-controlled free drive 
%
%   Outputs:
%       enable - A scalar value representing the enable state.
%                1 for an enabled parking maneuver, -1 for path following, and
%                0 for invalid maneuvers.

if maneuverType == 1        % Park Maneuver
    enable = 1;
elseif maneuverType == 3    % Path Following
    enable = -1;
else
    enable = 0;
    fprintf("Error occcured in ManeuverSwitch() - no valid manuever");
end

== matlab function s7_template_extra/Control Software/Determine Speed ==
  data: position_enable input; v output; pos input; vmax input
function v = SetSpeed(position_enable, pos, vmax)
% SetSpeed Selects speed based on position control enable status.
%
%   v = SetSpeed(position_enable, pos, vmax) returns 'pos' if 
%   position_enable is true (1), otherwise returns 'vmax'.
%
%   Inputs:
%       position_enable - Boolean flag indicating position control status.
%       pos - Speed to set when position control is enabled.
%       vmax - Maximum speed to set when position control is disabled.
%
%   Output:
%       v - The determined speed value [ m/s ].

if position_enable == 1
    v = pos;
else
    v = vmax;
end

== matlab function s7_template_extra/Control Software/Path Controller/Ref - Reference Signal Generator/MATLAB Function ==
  data: s_star output; psi_star output; breakslen input; points input; coefs input; periodic input; K_star output; s input size=2; v_star input; P_p_Tt parameter
function [s_star, psi_star, K_star] = GetReferenceTrack(breakslen, points, coefs, ...
    periodic, s, v_star, P_p_Tt)
% The guidance signal generator (parent subsystem) looks into the future to
% compensate for the vehicle's steering delay. It uses arc length to define a point
% on the desired trajectory curve that is ahead of the current position s.

% Inputs:
%   breakslen - Array of break lengths defining the spline segments.
%   points    - Array of points defining the spline path.
%   coefs     - Coefficients of the spline segments.
%   periodic  - Boolean indicating if the path is periodic (circular).
%   s         - Current position on the path.
%   v_star    - Desired speed of the vehicle [m/s].
%   P_p_Tt    - Time ahead to look on the path to compensate for delay [s].

% Outputs:
%   s_star    - Next point [s1_star, s2_star] on the reference path for path-following control.
%   psi_star  - Desired yaw angle at s_star [rad].
%   K_star    - Signed curvature at s_star.

% Function logic:
% The function calculates the closest point on the target trajectory to the vehicle's
% rear axle and the associated yaw angle and curvature, taking into account the vehicle's
% speed and the delay compensation parameter P_p_Tt.

[w, widx] = mbc_spline_get_reference(s, breakslen, points, ...
coefs, periodic, v_star, P_p_Tt);

psi_star = w(2);    % Desired yaw angle
K_star = w(5);      % Signed curvature
s_star = [w(3), w(4)]; % [s1_star, s2_star] Next point for path following control

end
